simulink model "TCS_straight"  (R2023a)
settings: Solver=VariableStepAuto  StartTime=0.0  StopTime=10.0  RelTol=1e-3
values from neighbouring files (symbols this model uses):
  T1 = 2,T2=2,alpha1=-1.8,alpha2=0.4,A=1    [abs_trial_second_version.m]
undefined symbols (not defined in the file or in its folder): A, alpha1, alpha2, T2, u1, u2, u3
settings Model: Creator=ycmxy  LastModifiedBy=Administrator
settings DebuggingCC: UnconnectedInputMsg=warning  UnconnectedOutputMsg=warning  UnconnectedLineMsg=warning
settings ModelReferenceCC: EnableRefExpFcnMdlSchedulingChecks=on
settings RTWCC: DLArmComputeVersion=19.05

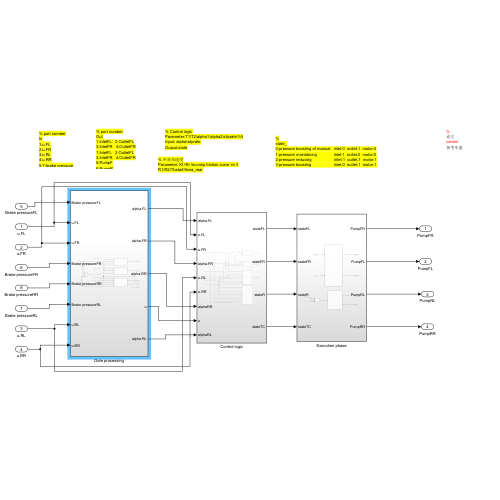
[thumbnail: Simulink's stored preview of the top-level diagram]
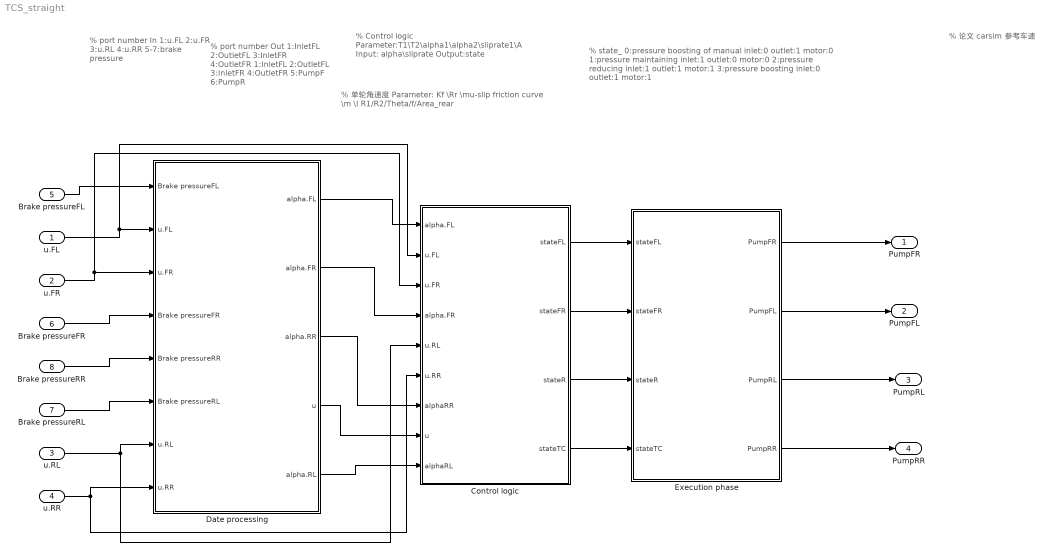
== system TCS_straight ==
  note: % 单轮角速度
      | Parameter: Kf \Rr \mu-slip friction curve \m \I
      | R1/R2/Theta/f/Area_rear
  note: % port number
      | In
      | 1:u.FL
      | 2:u.FR
      | 3:u.RL
      | 4:u.RR
      | 5-7:brake pressure
  note: % Control logic
      | Parameter:T1\T2\alpha1\alpha2\sliprate1\A
      | Input: alpha\sliprate
      | Output:state
  note: %
      | state_
      | 0:pressure boosting of manual inlet:0 outlet:1 motor:0
      | 1:pressure maintaining inlet:1 outlet:0 motor:0
      | 2:pressure reducing inlet:1 outlet:1 motor:1
      | 3:pressure boosting inlet:0 outlet:1 motor:1
  note: % port number
      | Out
      | 1:InletFL 2:OutletFL 3:InletFR 4:OutletFR
      | 1:InletFL 2:OutletFL
      | 3:InletFR 4:OutletFR
      | 5:PumpF
      | 6:PumpR
  note: %
      | 论文
      | carsim
      | 参考车速
  u.FL : Inport
  u.FR : Inport  Port=2
  u.RL : Inport  Port=3
  u.RR : Inport  Port=4
  Brake pressureFL : Inport  Port=5
  Brake pressureFR : Inport  Port=6
  Brake pressureRL : Inport  Port=7
  Brake pressureRR : Inport  Port=8
  Control logic : Subsystem
  Date processing : Subsystem
  Execution phase : Subsystem
  PumpFR : Outport  VectorParamsAs1DForOutWhenUnconnected=off
  PumpFL : Outport  Port=2  VectorParamsAs1DForOutWhenUnconnected=off
  PumpRL : Outport  Port=3  VectorParamsAs1DForOutWhenUnconnected=off
  PumpRR : Outport  Port=4  VectorParamsAs1DForOutWhenUnconnected=off
  wires:
  Execution phase/1(PumpFR) -> PumpFR/1
  u.RR/1 -> Date processing/8(u.RR), Control logic/6(u.RR)
  Brake pressureFL/1 -> Date processing/1(Brake pressureFL)
  Date processing/1(alpha.FL) -> Control logic/1(alpha.FL)
  u.FR/1 -> Control logic/3(u.FR), Date processing/3(u.FR)
  u.FL/1 -> Control logic/2(u.FL), Date processing/2(u.FL)
  Control logic/2(stateFR) -> Execution phase/2(stateFR)
  Date processing/2(alpha.FR) -> Control logic/4(alpha.FR)
  Execution phase/3(PumpRL) -> PumpRL/1
  Brake pressureFR/1 -> Date processing/4(Brake pressureFR)
  Control logic/3(stateR) -> Execution phase/3(stateR)
  Date processing/4(u) -> Control logic/8(u)
  Date processing/3(alpha.RR) -> Control logic/7(alphaRR)
  Brake pressureRR/1 -> Date processing/5(Brake pressureRR)
  u.RL/1 -> Control logic/5(u.RL), Date processing/7(u.RL)
  Control logic/1(stateFL) -> Execution phase/1(stateFL)
  Execution phase/4(PumpRR) -> PumpRR/1
  Brake pressureRL/1 -> Date processing/6(Brake pressureRL)
  Execution phase/2(PumpFL) -> PumpFL/1
  Date processing/5(alpha.RL) -> Control logic/9(alphaRL)
  Control logic/4(stateTC) -> Execution phase/4(stateTC)

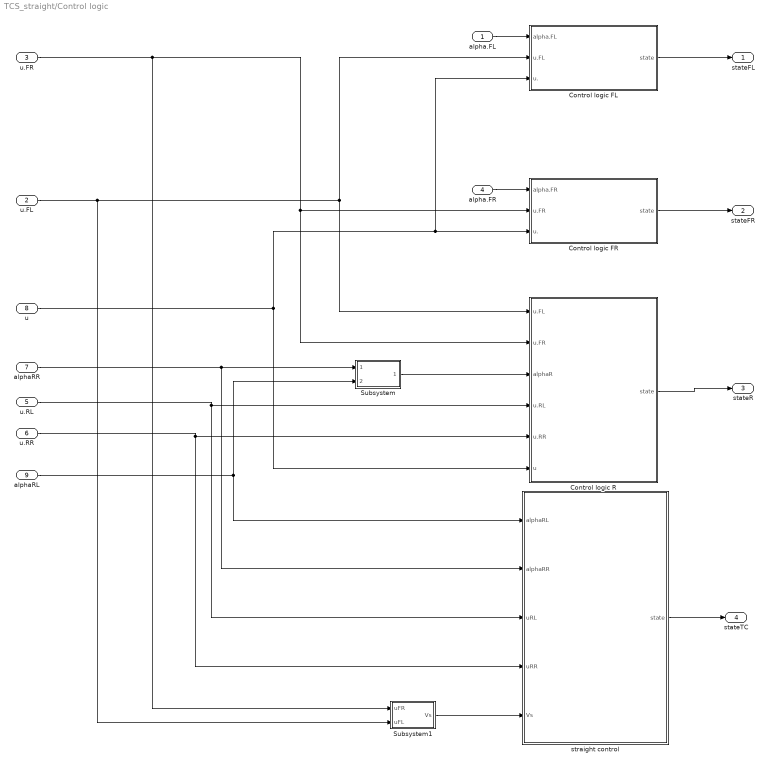
== system TCS_straight/Control logic ==
  alpha.FL : Inport
  u.FL : Inport  Port=2
  u.FR : Inport  Port=3
  alpha.FR : Inport  Port=4
  u.RL : Inport  Port=5
  u.RR : Inport  Port=6
  alphaRR : Inport  Port=7
  u : Inport  Port=8
  alphaRL : Inport  Port=9
  Control logic FL : Subsystem
  Control logic FR : Subsystem
  Control logic R : Subsystem
  Subsystem : Subsystem
  Subsystem1 : Subsystem
  straight control : Subsystem
  stateFL : Outport
  stateFR : Outport  Port=2
  stateR : Outport  Port=3
  stateTC : Outport  Port=4
  wires:
  u.FL/1 -> Subsystem1/2(uFL), Control logic FL/2(u.FL), Control logic R/1(u.FL)
  u.RR/1 -> straight control/4(uRR), Control logic R/5(u.RR)
  Control logic FR/1(state) -> stateFR/1
  u.FR/1 -> Subsystem1/1(uFR), Control logic R/2(u.FR), Control logic FR/2(u.FR)
  alpha.FR/1 -> Control logic FR/1(alpha.FR)
  alpha.FL/1 -> Control logic FL/1(alpha.FL)
  Control logic R/1(state) -> stateR/1
  Control logic FL/1(state) -> stateFL/1
  u.RL/1 -> straight control/3(uRL), Control logic R/4(u.RL)
  u/1 -> Control logic FR/3(u.), Control logic FL/3(u.), Control logic R/6(u)
  alphaRR/1 -> straight control/2(alphaRR), Subsystem/1(alphaRR)
  alphaRL/1 -> straight control/1(alphaRL), Subsystem/2(alphaRL)
  Subsystem/1(alphaR) -> Control logic R/3(alphaR)
  Subsystem1/1(Vs) -> straight control/5(Vs)
  straight control/1(state) -> stateTC/1

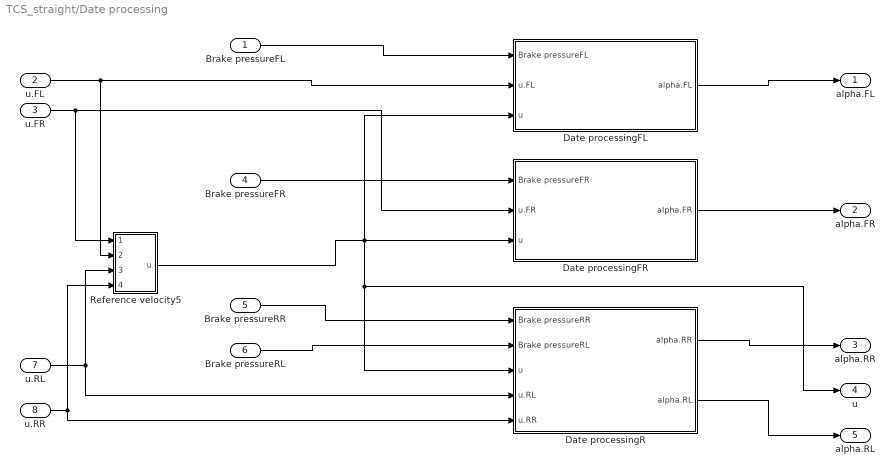
== system TCS_straight/Date processing ==
  Brake pressureFL : Inport
  u.FL : Inport  Port=2
  u.FR : Inport  Port=3
  Brake pressureFR : Inport  Port=4
  Brake pressureRR : Inport  Port=5
  Brake pressureRL : Inport  Port=6
  u.RL : Inport  Port=7
  u.RR : Inport  Port=8
  Date processingFL : Subsystem
  Date processingFR : Subsystem
  Date processingR : Subsystem
  Reference velocity5 : Subsystem
  alpha.FL : Outport
  alpha.FR : Outport  Port=2
  alpha.RR : Outport  Port=3
  u : Outport  Port=4
  alpha.RL : Outport  Port=5
  wires:
  Date processingR/1(alpha.RR) -> alpha.RR/1
  u.FL/1 -> Reference velocity5/2(u.FL), Date processingFL/2(u.FL)
  Brake pressureRR/1 -> Date processingR/1(Brake pressureRR)
  u.FR/1 -> Reference velocity5/1(u.FR), Date processingFR/2(u.FR)
  Brake pressureFL/1 -> Date processingFL/1(Brake pressureFL)
  u.RL/1 -> Reference velocity5/3(u.RL), Date processingR/4(u.RL)
  Date processingFL/1(alpha.FL) -> alpha.FL/1
  Date processingFR/1(alpha.FR) -> alpha.FR/1
  Brake pressureFR/1 -> Date processingFR/1(Brake pressureFR)
  Brake pressureRL/1 -> Date processingR/2(Brake pressureRL)
  u.RR/1 -> Reference velocity5/4(u.RR), Date processingR/5(u.RR)
  Reference velocity5/1(u) -> Date processingFL/3(u), Date processingFR/3(u), u/1, Date processingR/3(u)
  Date processingR/2(alpha.RL) -> alpha.RL/1

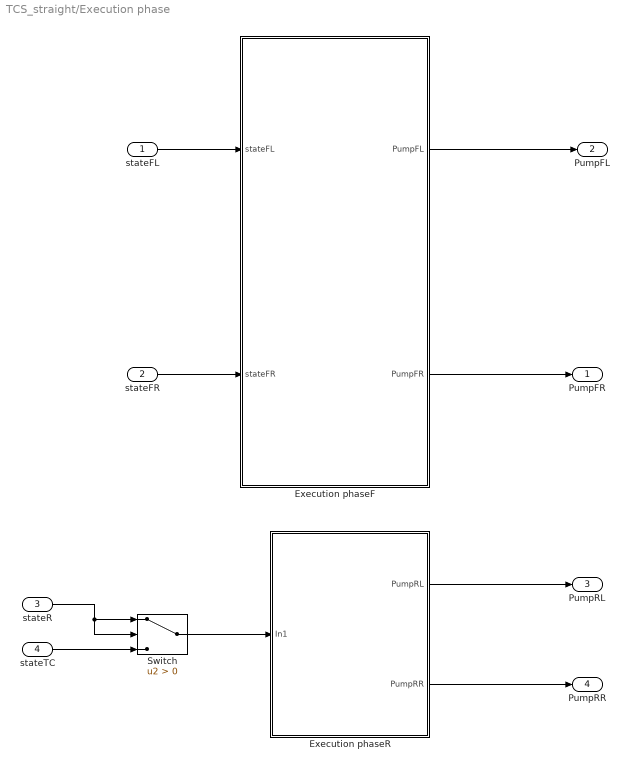
== system TCS_straight/Execution phase ==
  stateFL : Inport
  stateFR : Inport  Port=2
  stateR : Inport  Port=3
  stateTC : Inport  Port=4
  Execution phaseF : Subsystem
  Execution phaseR : Subsystem
  Switch : Switch  Criteria=u2 > Threshold  SaturateOnIntegerOverflow=off  InputSameDT=off
  PumpFR : Outport
  PumpFL : Outport  Port=2
  PumpRL : Outport  Port=3
  PumpRR : Outport  Port=4
  wires:
  stateFL/1 -> Execution phaseF/1(stateFL)
  stateFR/1 -> Execution phaseF/2(stateFR)
  Execution phaseR/1(PumpRL) -> PumpRL/1
  Execution phaseF/1(PumpFL) -> PumpFL/1
  Execution phaseF/2(PumpFR) -> PumpFR/1
  Execution phaseR/2(PumpRR) -> PumpRR/1
  stateR/1 -> Switch/1, Switch/2
  stateTC/1 -> Switch/3
  Switch/1 -> Execution phaseR/1(In1)

== system TCS_straight/Control logic/Control logic FL ==
  alpha.FL : Inport
  u.FL : Inport  Port=2
  u. : Inport  Port=3
  FL : Stateflow chart  TreatAsAtomicUnit=on
  Gain : Gain  Gain=0.8
  state : Outport  VectorParamsAs1DForOutWhenUnconnected=off
  wires:
  alpha.FL/1 -> FL/1(alpha)
  FL/1(state) -> state/1
  u.FL/1 -> FL/2(omegaR)
  Gain/1 -> FL/3(sliprate1)
  u./1 -> Gain/1

== system TCS_straight/Control logic/Control logic FR ==
  alpha.FR : Inport
  u.FR : Inport  Port=2
  u. : Inport  Port=3
  FR : Stateflow chart  TreatAsAtomicUnit=on
  Gain : Gain  Gain=0.8
  state : Outport  VectorParamsAs1DForOutWhenUnconnected=off
  wires:
  alpha.FR/1 -> FR/1(alpha)
  FR/1(state) -> state/1
  u.FR/1 -> FR/2(omegaR)
  Gain/1 -> FR/3(sliprate1)
  u./1 -> Gain/1

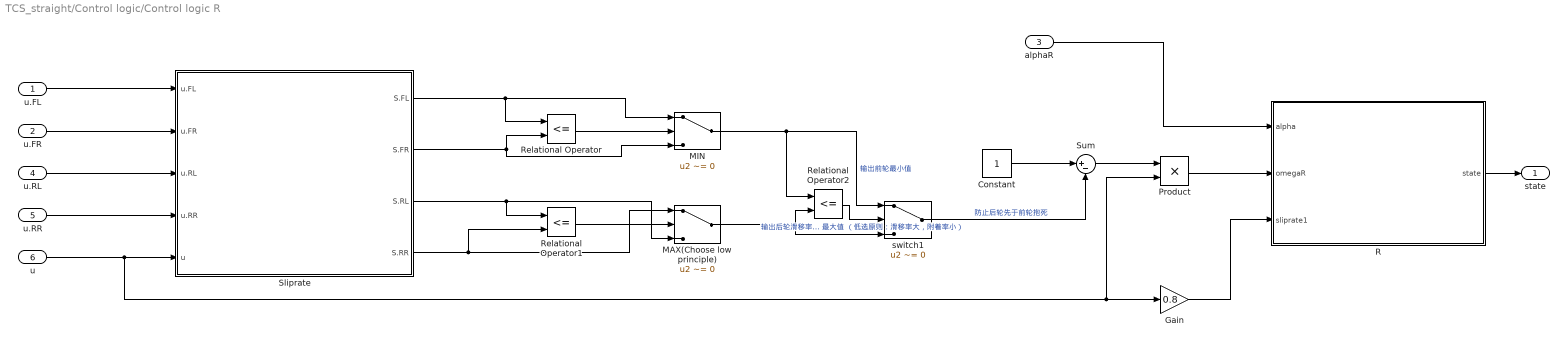
== system TCS_straight/Control logic/Control logic R ==
  u.FL : Inport
  u.FR : Inport  Port=2
  alphaR : Inport  Port=3
  u.RL : Inport  Port=4
  u.RR : Inport  Port=5
  u : Inport  Port=6
  Constant : Constant
  Gain : Gain  Gain=0.8
  MAX(Choose low principle) : Switch  Criteria=u2 ~= 0  SaturateOnIntegerOverflow=off  InputSameDT=off
  MIN : Switch  Criteria=u2 ~= 0  SaturateOnIntegerOverflow=off  InputSameDT=off
  Product : Product
  R : Stateflow chart  TreatAsAtomicUnit=on
  Relational Operator : RelationalOperator  Operator=<=  OutDataTypeStr=boolean  RndMeth=Simplest  InputSameDT=off
  Relational Operator1 : RelationalOperator  Operator=<=  OutDataTypeStr=boolean  RndMeth=Simplest  InputSameDT=off
  Relational Operator2 : RelationalOperator  Operator=<=  OutDataTypeStr=boolean  RndMeth=Simplest  InputSameDT=off
  Sliprate : Subsystem
  Sum : Sum  Inputs=|+-
  switch1 : Switch  Criteria=u2 ~= 0  SaturateOnIntegerOverflow=off  InputSameDT=off
  state : Outport  VectorParamsAs1DForOutWhenUnconnected=off
  wires:
  MAX(Choose low principle)/1 -> switch1/3, Relational Operator2/2  "输出后轮滑移率 最大值 （低选原则：滑移率大，附着率小）"
  switch1/1 -> Sum/2  "防止后轮先于前轮抱死"
  u.FR/1 -> Sliprate/2(u.FR)
  Sliprate/2(S.FR) -> MIN/3, Relational Operator/2
  Sliprate/1(S.FL) -> Relational Operator/1, MIN/1
  Relational Operator2/1 -> switch1/2
  Relational Operator/1 -> MIN/2
  MIN/1 -> Relational Operator2/1, switch1/1  "输出前轮最小值"
  Sliprate/4(S.RR) -> MAX(Choose low principle)/1, Relational Operator1/2
  Relational Operator1/1 -> MAX(Choose low principle)/2
  u.RL/1 -> Sliprate/3(u.RL)
  Sliprate/3(S.RL) -> Relational Operator1/1, MAX(Choose low principle)/3
  u/1 -> Product/2, Gain/1, Sliprate/5(u)
  alphaR/1 -> R/1(alpha)
  u.FL/1 -> Sliprate/1(u.FL)
  R/1(state) -> state/1
  u.RR/1 -> Sliprate/4(u.RR)
  Gain/1 -> R/3(sliprate1)
  Constant/1 -> Sum/1
  Product/1 -> R/2(omegaR)
  Sum/1 -> Product/1

== system TCS_straight/Control logic/Subsystem ==
  alphaRR : Inport
  alphaRL : Inport  Port=2
  Multiply : Gain  Gain=1/2
  Sum : Sum  Inputs=|++
  alphaR : Outport
  wires:
  alphaRR/1 -> Sum/1
  alphaRL/1 -> Sum/2
  Sum/1 -> Multiply/1
  Multiply/1 -> alphaR/1

== system TCS_straight/Control logic/Subsystem1 ==
  uFR : Inport
  uFL : Inport  Port=2
  Multiply : Gain  Gain=1/2
  Sum : Sum  Inputs=|++
  Vs : Outport
  wires:
  uFR/1 -> Sum/1
  uFL/1 -> Sum/2
  Sum/1 -> Multiply/1
  Multiply/1 -> Vs/1

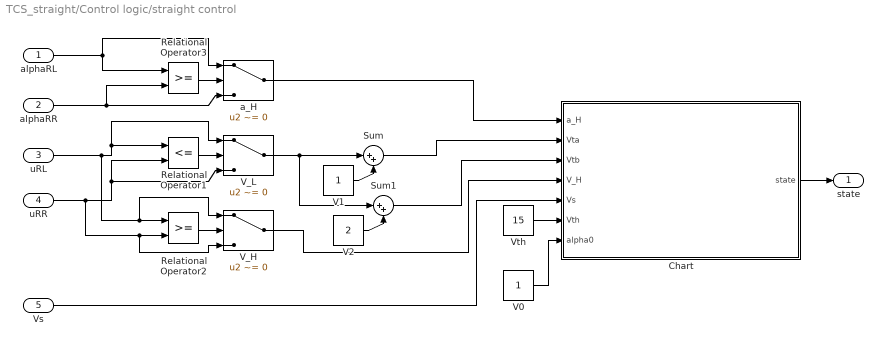
== system TCS_straight/Control logic/straight control ==
  alphaRL : Inport
  alphaRR : Inport  Port=2
  uRL : Inport  Port=3
  uRR : Inport  Port=4
  Vs : Inport  Port=5
  Chart : Stateflow chart  TreatAsAtomicUnit=on
  Relational Operator1 : RelationalOperator  Operator=<=  OutDataTypeStr=boolean  RndMeth=Simplest  InputSameDT=off
  Relational Operator2 : RelationalOperator  OutDataTypeStr=boolean  RndMeth=Simplest  InputSameDT=off
  Relational Operator3 : RelationalOperator  OutDataTypeStr=boolean  RndMeth=Simplest  InputSameDT=off
  Sum : Sum  Inputs=|++
  Sum1 : Sum  Inputs=|++
  V0 : Constant
  V1 : Constant
  V2 : Constant  Value=2
  V_H : Switch  Criteria=u2 ~= 0  SaturateOnIntegerOverflow=off  InputSameDT=off
  V_L : Switch  Criteria=u2 ~= 0  SaturateOnIntegerOverflow=off  InputSameDT=off
  Vth : Constant  Value=15
  a_H : Switch  Criteria=u2 ~= 0  SaturateOnIntegerOverflow=off  InputSameDT=off
  state : Outport
  wires:
  Relational Operator3/1 -> a_H/2
  alphaRL/1 -> Relational Operator3/1, a_H/1
  alphaRR/1 -> a_H/3, Relational Operator3/2
  Relational Operator1/1 -> V_L/2
  uRL/1 -> V_H/1, Relational Operator2/1, V_L/1, Relational Operator1/1
  uRR/1 -> V_H/3, Relational Operator2/2, V_L/3, Relational Operator1/2
  Relational Operator2/1 -> V_H/2
  V1/1 -> Sum/2
  V_L/1 -> Sum/1, Sum1/1
  V2/1 -> Sum1/2
  Sum/1 -> Chart/2(Vta)
  Sum1/1 -> Chart/3(Vtb)
  Vs/1 -> Chart/5(Vs)
  V_H/1 -> Chart/4(V_H)
  a_H/1 -> Chart/1(a_H)
  Chart/1(state) -> state/1
  Vth/1 -> Chart/6(Vth)
  V0/1 -> Chart/7(alpha0)

== system TCS_straight/Date processing/Date processingFL ==
  Brake pressureFL : Inport
  u.FL : Inport  Port=2
  u : Inport  Port=3
  Tire angular velocity.FL : Subsystem
  alpha.FL : Outport
  wires:
  Tire angular velocity.FL/1(alpha.FL) -> alpha.FL/1
  u/1 -> Tire angular velocity.FL/3(u)
  Brake pressureFL/1 -> Tire angular velocity.FL/1(Brakepressure)
  u.FL/1 -> Tire angular velocity.FL/2(u.FL)

== system TCS_straight/Date processing/Date processingFR ==
  Brake pressureFR : Inport
  u.FR : Inport  Port=2
  u : Inport  Port=3
  Tire angular velocity.FR : Subsystem
  alpha.FR : Outport
  wires:
  u.FR/1 -> Tire angular velocity.FR/1(u.FR)
  Tire angular velocity.FR/1(alpha.FR) -> alpha.FR/1
  Brake pressureFR/1 -> Tire angular velocity.FR/3(Brake pressure)
  u/1 -> Tire angular velocity.FR/2(u)

== system TCS_straight/Date processing/Date processingR ==
  Brake pressureRR : Inport
  Brake pressureRL : Inport  Port=2
  u : Inport  Port=3
  u.RL : Inport  Port=4
  u.RR : Inport  Port=5
  Tire angular velocity.R : Subsystem
  Tire angular velocity.R1 : Subsystem
  alpha.RR : Outport
  alpha.RL : Outport  Port=2
  wires:
  Tire angular velocity.R/1(alpha.RR) -> alpha.RR/1
  u.RR/1 -> Tire angular velocity.R/3(u.RR)
  Brake pressureRR/1 -> Tire angular velocity.R/1(Brake pressureRR)
  Tire angular velocity.R1/1(alpha.RR) -> alpha.RL/1
  u/1 -> Tire angular velocity.R/2(u), Tire angular velocity.R1/2(u)
  u.RL/1 -> Tire angular velocity.R1/3(u.RL)
  Brake pressureRL/1 -> Tire angular velocity.R1/1(Brake pressureRR)

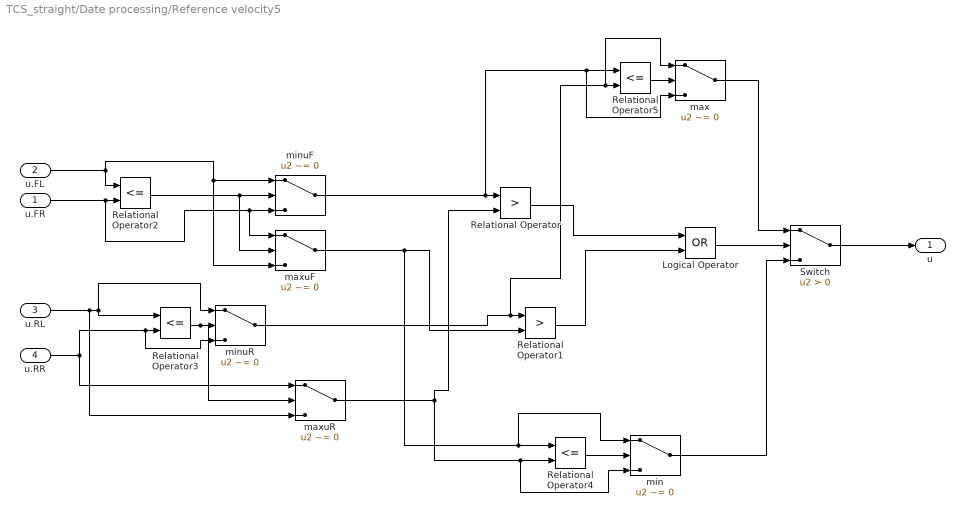
== system TCS_straight/Date processing/Reference velocity5 ==
  u.FR : Inport
  u.FL : Inport  Port=2
  u.RL : Inport  Port=3
  u.RR : Inport  Port=4
  Logical Operator : Logic  Operator=OR  AllPortsSameDT=off  OutDataTypeStr=boolean
  Relational Operator : RelationalOperator  Operator=>  OutDataTypeStr=boolean  RndMeth=Simplest  InputSameDT=off
  Relational Operator1 : RelationalOperator  Operator=>  OutDataTypeStr=boolean  RndMeth=Simplest  InputSameDT=off
  Relational Operator{2..5} (4 alike) : RelationalOperator  Operator=<=  OutDataTypeStr=boolean  RndMeth=Simplest  InputSameDT=off
  Switch : Switch  Criteria=u2 > Threshold  SaturateOnIntegerOverflow=off  InputSameDT=off
  max : Switch  Criteria=u2 ~= 0  SaturateOnIntegerOverflow=off  InputSameDT=off
  maxuF : Switch  Criteria=u2 ~= 0  SaturateOnIntegerOverflow=off  InputSameDT=off
  maxuR : Switch  Criteria=u2 ~= 0  SaturateOnIntegerOverflow=off  InputSameDT=off
  min : Switch  Criteria=u2 ~= 0  SaturateOnIntegerOverflow=off  InputSameDT=off
  minuF : Switch  Criteria=u2 ~= 0  SaturateOnIntegerOverflow=off  InputSameDT=off
  minuR : Switch  Criteria=u2 ~= 0  SaturateOnIntegerOverflow=off  InputSameDT=off
  u : Outport  VectorParamsAs1DForOutWhenUnconnected=off
  wires:
  u.FR/1 -> maxuF/1, minuF/3, Relational Operator2/2
  u.FL/1 -> minuF/1, maxuF/3, Relational Operator2/1
  u.RL/1 -> maxuR/3, minuR/1, Relational Operator3/1
  u.RR/1 -> maxuR/1, minuR/3, Relational Operator3/2
  minuF/1 -> max/3, Relational Operator5/1, Relational Operator/1
  maxuR/1 -> min/3, Relational Operator4/2, Relational Operator/2
  minuR/1 -> max/1, Relational Operator5/2, Relational Operator1/1
  maxuF/1 -> min/1, Relational Operator4/1, Relational Operator1/2
  Relational Operator/1 -> Logical Operator/1
  Relational Operator1/1 -> Logical Operator/2
  Logical Operator/1 -> Switch/2
  min/1 -> Switch/3
  max/1 -> Switch/1
  Switch/1 -> u/1
  Relational Operator2/1 -> minuF/2, maxuF/2
  Relational Operator3/1 -> maxuR/2, minuR/2
  Relational Operator4/1 -> min/2
  Relational Operator5/1 -> max/2

== system TCS_straight/Execution phase/Execution phaseF ==
  stateFL : Inport
  stateFR : Inport  Port=2
  Execution phaseFL : Stateflow chart  TreatAsAtomicUnit=on
  Execution phaseFR : Stateflow chart  TreatAsAtomicUnit=on
  PumpFL : Outport  VectorParamsAs1DForOutWhenUnconnected=off
  PumpFR : Outport  Port=2  VectorParamsAs1DForOutWhenUnconnected=off
  wires:
  stateFL/1 -> Execution phaseFL/1(state)
  stateFR/1 -> Execution phaseFR/1(state)
  Execution phaseFL/1(Pump) -> PumpFL/1
  Execution phaseFR/1(Pump) -> PumpFR/1

== system TCS_straight/Execution phase/Execution phaseR ==
  In1 : Inport
  Execution phaseRL : Stateflow chart  TreatAsAtomicUnit=on
  Execution phaseRR : Stateflow chart  TreatAsAtomicUnit=on
  PumpRL : Outport  VectorParamsAs1DForOutWhenUnconnected=off
  PumpRR : Outport  Port=2  VectorParamsAs1DForOutWhenUnconnected=off
  wires:
  In1/1 -> Execution phaseRR/1(state), Execution phaseRL/1(state)
  Execution phaseRR/1(Pump) -> PumpRR/1
  Execution phaseRL/1(Pump) -> PumpRL/1

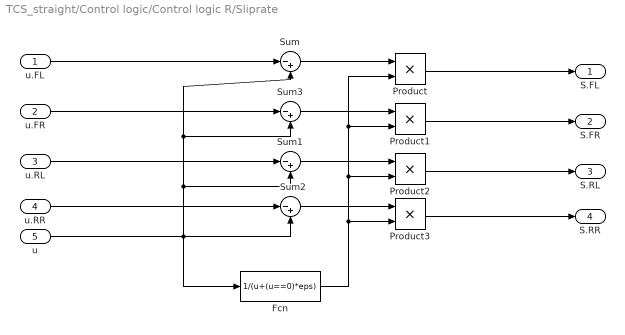
== system TCS_straight/Control logic/Control logic R/Sliprate ==
  u.FL : Inport
  u.FR : Inport  Port=2
  u.RL : Inport  Port=3
  u.RR : Inport  Port=4
  u : Inport  Port=5
  Fcn : Fcn  Expr=1/(u+(u==0)*eps)
  Product{,1..3} (4 alike) : Product
  Sum{,1..3} (4 alike) : Sum  Inputs=|-+
  S.FL : Outport  VectorParamsAs1DForOutWhenUnconnected=off
  S.FR : Outport  Port=2  VectorParamsAs1DForOutWhenUnconnected=off
  S.RL : Outport  Port=3  VectorParamsAs1DForOutWhenUnconnected=off
  S.RR : Outport  Port=4  VectorParamsAs1DForOutWhenUnconnected=off
  wires:
  Sum2/1 -> Product3/1
  Sum/1 -> Product/1
  Fcn/1 -> Product3/2, Product2/2, Product1/2, Product/2
  Sum1/1 -> Product2/1
  Sum3/1 -> Product1/1
  u/1 -> Sum2/2, Fcn/1, Sum1/2, Sum3/2, Sum/2
  u.RL/1 -> Sum1/1
  u.RR/1 -> Sum2/1
  Product2/1 -> S.RL/1
  Product3/1 -> S.RR/1
  Product/1 -> S.FL/1
  Product1/1 -> S.FR/1
  u.FL/1 -> Sum/1
  u.FR/1 -> Sum3/1

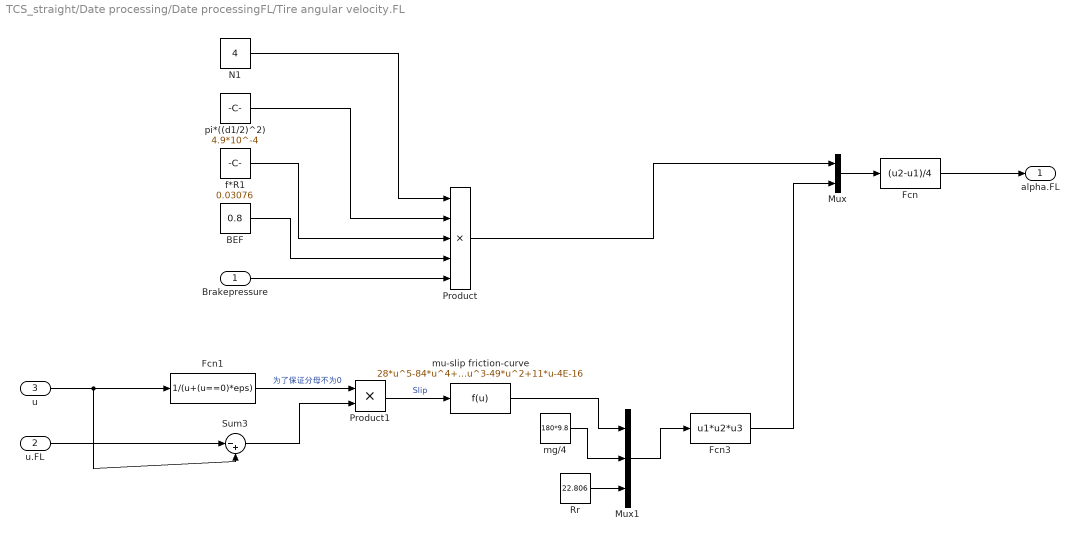
== system TCS_straight/Date processing/Date processingFL/Tire angular velocity.FL ==
  Brakepressure : Inport
  u.FL : Inport  Port=2
  u : Inport  Port=3
  BEF : Constant  Value=0.8
  Fcn : Fcn  Expr=(u2-u1)/4
  Fcn1 : Fcn  Expr=1/(u+(u==0)*eps)
  Fcn3 : Fcn  Expr=u1*u2*u3
  Mux : Mux  Inputs=2
  Mux1 : Mux  Inputs=3
  N1 : Constant  Value=4
  Product : Product  Inputs=5
  Product1 : Product
  Rr : Constant  Value=22.806
  Sum3 : Sum  Inputs=|-+
  f*R1 : Constant  Value=0.03076
  mg/4 : Constant  Value=180*9.8
  mu-slip friction-curve : Fcn  Expr=28*u^5-84*u^4+94.5*u^3-49*u^2+11*u-4E-16
  pi*((d1/2)^2) : Constant  Value=4.9*10^-4
  alpha.FL : Outport  VectorParamsAs1DForOutWhenUnconnected=off
  wires:
  mu-slip friction-curve/1 -> Mux1/1
  Sum3/1 -> Product1/2
  u.FL/1 -> Sum3/1
  u/1 -> Fcn1/1, Sum3/2
  Fcn1/1 -> Product1/1  "为了保证分母不为0"
  Product1/1 -> mu-slip friction-curve/1  "Slip"
  N1/1 -> Product/1
  pi*((d1/2)^2)/1 -> Product/2
  f*R1/1 -> Product/3
  BEF/1 -> Product/4
  Brakepressure/1 -> Product/5
  Mux/1 -> Fcn/1
  Product/1 -> Mux/1
  Fcn/1 -> alpha.FL/1
  Mux1/1 -> Fcn3/1
  mg/4/1 -> Mux1/2
  Rr/1 -> Mux1/3
  Fcn3/1 -> Mux/2

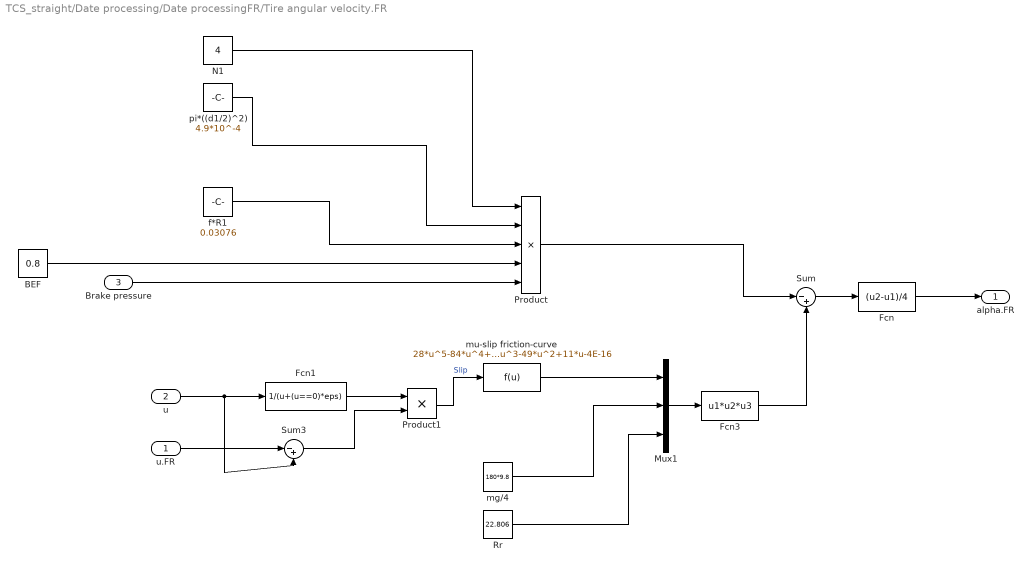
== system TCS_straight/Date processing/Date processingFR/Tire angular velocity.FR ==
  u.FR : Inport
  u : Inport  Port=2
  Brake pressure : Inport  Port=3
  BEF : Constant  Value=0.8
  Fcn : Fcn  Expr=(u2-u1)/4
  Fcn1 : Fcn  Expr=1/(u+(u==0)*eps)
  Fcn3 : Fcn  Expr=u1*u2*u3
  Mux1 : Mux  Inputs=3
  N1 : Constant  Value=4
  Product : Product  Inputs=5
  Product1 : Product
  Rr : Constant  Value=22.806
  Sum : Sum  Inputs=|-+
  Sum3 : Sum  Inputs=|-+
  f*R1 : Constant  Value=0.03076
  mg/4 : Constant  Value=180*9.8
  mu-slip friction-curve : Fcn  Expr=28*u^5-84*u^4+94.5*u^3-49*u^2+11*u-4E-16
  pi*((d1/2)^2) : Constant  Value=4.9*10^-4
  alpha.FR : Outport  VectorParamsAs1DForOutWhenUnconnected=off
  wires:
  Fcn1/1 -> Product1/1
  u/1 -> Fcn1/1, Sum3/2
  u.FR/1 -> Sum3/1
  Sum3/1 -> Product1/2
  Sum/1 -> Fcn/1
  BEF/1 -> Product/4
  f*R1/1 -> Product/3
  pi*((d1/2)^2)/1 -> Product/2
  N1/1 -> Product/1
  Brake pressure/1 -> Product/5
  Product/1 -> Sum/1
  Fcn3/1 -> Sum/2
  Mux1/1 -> Fcn3/1
  mu-slip friction-curve/1 -> Mux1/1
  Product1/1 -> mu-slip friction-curve/1  "Slip"
  mg/4/1 -> Mux1/2
  Rr/1 -> Mux1/3
  Fcn/1 -> alpha.FR/1

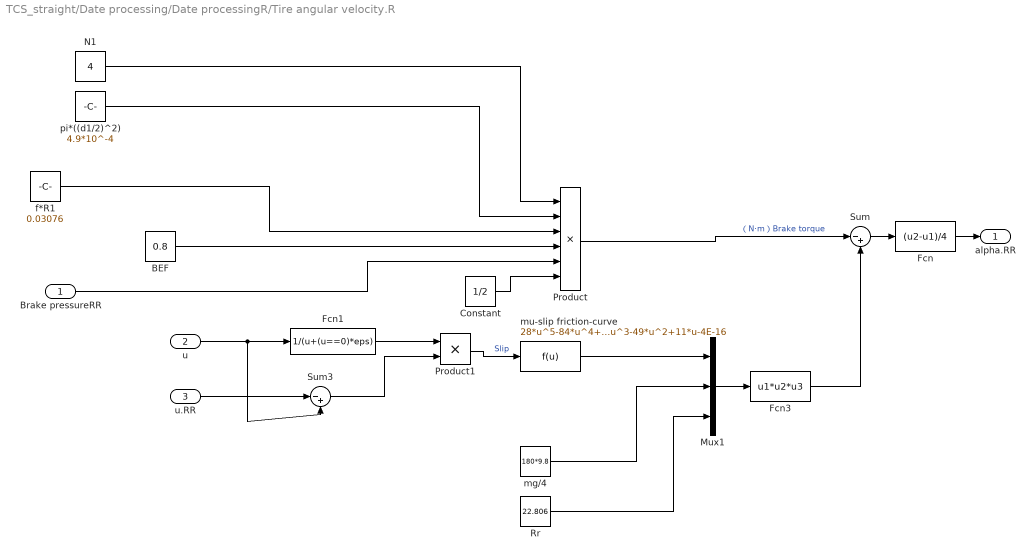
== system TCS_straight/Date processing/Date processingR/Tire angular velocity.R ==
  Brake pressureRR : Inport
  u : Inport  Port=2
  u.RR : Inport  Port=3
  BEF : Constant  Value=0.8
  Constant : Constant  Value=1/2
  Fcn : Fcn  Expr=(u2-u1)/4
  Fcn1 : Fcn  Expr=1/(u+(u==0)*eps)
  Fcn3 : Fcn  Expr=u1*u2*u3
  Mux1 : Mux  Inputs=3
  N1 : Constant  Value=4
  Product : Product  Inputs=6
  Product1 : Product
  Rr : Constant  Value=22.806
  Sum : Sum  Inputs=|-+
  Sum3 : Sum  Inputs=|-+
  f*R1 : Constant  Value=0.03076
  mg/4 : Constant  Value=180*9.8
  mu-slip friction-curve : Fcn  Expr=28*u^5-84*u^4+94.5*u^3-49*u^2+11*u-4E-16
  pi*((d1/2)^2) : Constant  Value=4.9*10^-4
  alpha.RR : Outport  VectorParamsAs1DForOutWhenUnconnected=off
  wires:
  Sum3/1 -> Product1/2
  u.RR/1 -> Sum3/1
  u/1 -> Sum3/2, Fcn1/1
  Fcn1/1 -> Product1/1
  Product/1 -> Sum/1  "（N·m）Brake torque"
  BEF/1 -> Product/4
  N1/1 -> Product/1
  f*R1/1 -> Product/3
  pi*((d1/2)^2)/1 -> Product/2
  Brake pressureRR/1 -> Product/5
  Constant/1 -> Product/6
  Sum/1 -> Fcn/1
  Fcn/1 -> alpha.RR/1
  mu-slip friction-curve/1 -> Mux1/1
  Mux1/1 -> Fcn3/1
  mg/4/1 -> Mux1/2
  Product1/1 -> mu-slip friction-curve/1  "Slip"
  Rr/1 -> Mux1/3
  Fcn3/1 -> Sum/2

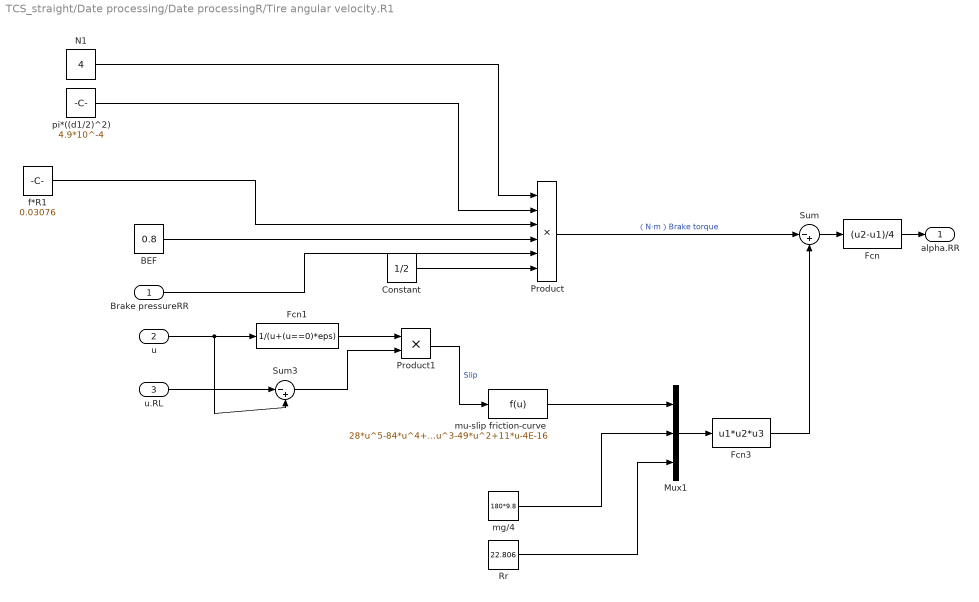
== system TCS_straight/Date processing/Date processingR/Tire angular velocity.R1 ==
  Brake pressureRR : Inport
  u : Inport  Port=2
  u.RL : Inport  Port=3
  BEF : Constant  Value=0.8
  Constant : Constant  Value=1/2
  Fcn : Fcn  Expr=(u2-u1)/4
  Fcn1 : Fcn  Expr=1/(u+(u==0)*eps)
  Fcn3 : Fcn  Expr=u1*u2*u3
  Mux1 : Mux  Inputs=3
  N1 : Constant  Value=4
  Product : Product  Inputs=6
  Product1 : Product
  Rr : Constant  Value=22.806
  Sum : Sum  Inputs=|-+
  Sum3 : Sum  Inputs=|-+
  f*R1 : Constant  Value=0.03076
  mg/4 : Constant  Value=180*9.8
  mu-slip friction-curve : Fcn  Expr=28*u^5-84*u^4+94.5*u^3-49*u^2+11*u-4E-16
  pi*((d1/2)^2) : Constant  Value=4.9*10^-4
  alpha.RR : Outport  VectorParamsAs1DForOutWhenUnconnected=off
  wires:
  Sum3/1 -> Product1/2
  u.RL/1 -> Sum3/1
  u/1 -> Sum3/2, Fcn1/1
  Fcn1/1 -> Product1/1
  N1/1 -> Product/1
  Product/1 -> Sum/1  "（N·m）Brake torque"
  pi*((d1/2)^2)/1 -> Product/2
  f*R1/1 -> Product/3
  BEF/1 -> Product/4
  Constant/1 -> Product/6
  Brake pressureRR/1 -> Product/5
  Rr/1 -> Mux1/3
  mu-slip friction-curve/1 -> Mux1/1
  Mux1/1 -> Fcn3/1
  mg/4/1 -> Mux1/2
  Fcn3/1 -> Sum/2
  Product1/1 -> mu-slip friction-curve/1  "Slip"
  Sum/1 -> Fcn/1
  Fcn/1 -> alpha.RR/1

== stateflow chart TCS_straight/Control logic/Control logic R/R ==
  state state_ [group]
    0:pressure boosting of manual
    1:pressure maintaining
    2:pressure reducing
    3:pressure boosting
    Parameter:
    T1 T2
    alpha1\alpha2\sliprate1\A
    Input: alpha\sliprate
    Output:state
  state phase2     %state pressure reducing
    state phase3_1
      en:
      state= 2;
    state phase3_2
      en:
      state= 1;
    (default) -> phase3_1
    phase3_1 -> phase3_2 : after(T1,sec)
    phase3_2 -> phase3_1 : after(T1,sec)
  state phase0
    en:
    state= 0;
  state phase1
    en:
    state= 1;
  state phase4_2     %state pressure reducing
    state phase4_2_1
      en:
      state= 2;
    state phase4_2_2
      en:
      state= 1;
    (default) -> phase4_2_1
    phase4_2_1 -> phase4_2_2 : after(T1,sec)
    phase4_2_2 -> phase4_2_1 : after(T1,sec)
  state phase4_1     %state pressure boosting
    state phase4_1_1
      en:
      state= 3;
    state phase4_1_2
      en:
      state= 1;
    (default) -> phase4_1_1
    phase4_1_1 -> phase4_1_2 : after(T2,sec)
    phase4_1_2 -> phase4_1_1 : after(T2,sec)
  state phase3
    en:
    state= 1;
  state phase4_ 1 2 3: [group]
    路面附着系数识别阶段
  state phase4_3
    en:
    state= 1;
  state phase5     %state pressure boosting
    state phase5_1
      en:
      state= 3;
    state phase5_2
      en:
      state= 1;
    (default) -> phase5_1
    phase5_1 -> phase5_2 : after(T2,sec)
    phase5_2 -> phase5_1 : after(T2,sec)
  state phase5_ [group]
    第一周期结束
  (default) -> phase0
  phase0 -> phase1 : [alpha<alpha1]
      | %开始作用
  phase1 -> phase2     %state pressure reducing : [omegaR<sliprate1]
  phase5     %state pressure boosting -> phase1 : [alpha<alpha1]
  phase2     %state pressure reducing -> phase3 : [alpha>alpha1]
  phase3 -> (junction 25)
  (junction 25) -> phase4_1     %state pressure boosting [order 3] : [alpha>A]
  (junction 25) -> phase4_2     %state pressure reducing [order 2] : [alpha<alpha2]
  (junction 25) -> phase4_3 [order 1] : [alpha2<alpha<A]
  phase4_2     %state pressure reducing -> phase4_3 : [alpha>alpha2]
  phase4_1     %state pressure boosting -> phase4_3 : [alpha<A]
  phase4_3 -> phase5     %state pressure boosting : [alpha<alpha2]
  data: alpha input; alpha1 parameter; alpha2 parameter; omegaR input; A parameter; T1 parameter; T2 parameter; state output; sliprate1 input

== stateflow chart TCS_straight/Control logic/Control logic FL/FL ==
  state state_ [group]
    0:pressure boosting of manual
    1:pressure maintaining
    2:pressure reducing
    3:pressure boosting
    Parameter:
    T1 T2
    alpha1\alpha2\sliprate1\A
    Input: alpha\sliprate
    Output:state
  state phase2     %state pressure reducing
    state phase2_1
      en:
      state= 2;
    state phase2_2
      en:
      state= 1;
    (default) -> phase2_1
    phase2_1 -> phase2_2 : after(T1,sec)
    phase2_2 -> phase2_1 : after(T1,sec)
  state phase0
    en:
    state= 0;
  state phase1
    en:
    state= 1;
  state phase4_2     %state pressure reducing
    state phase4_2_1
      en:
      state= 2;
    state phase4_2_2
      en:
      state= 1;
    (default) -> phase4_2_1
    phase4_2_1 -> phase4_2_2 : after(T1,sec)
    phase4_2_2 -> phase4_2_1 : after(T1,sec)
  state phase4_1     %state pressure boosting
    state phase4_1_1
      en:
      state= 3;
    state phase4_1_2
      en:
      state= 1;
    (default) -> phase4_1_1
    phase4_1_1 -> phase4_1_2 : after(T2,sec)
    phase4_1_2 -> phase4_1_1 : after(T2,sec)
  state phase3
    en:
    state= 1;
  state phase4_ 1 2 3: [group]
    路面附着系数识别阶段
  state phase4_3
    en:
    state= 1;
  state phase5     %state pressure boosting
    state phase5_1
      en:
      state= 3;
    state phase5_2
      en:
      state= 1;
    (default) -> phase5_1
    phase5_1 -> phase5_2 : after(T2,sec)
    phase5_2 -> phase5_1 : after(T2,sec)
  state phase5_ [group]
    第一周期结束
  (default) -> phase0
  phase0 -> phase1 : [alpha<alpha1]
      | %开始作用
  phase1 -> phase2     %state pressure reducing : [omegaR<sliprate1]
  phase5     %state pressure boosting -> phase1 : [alpha<alpha1]
  phase2     %state pressure reducing -> phase3 : [alpha>alpha1]
  phase3 -> (junction 25)
  (junction 25) -> phase4_1     %state pressure boosting [order 3] : [alpha>A]
  (junction 25) -> phase4_2     %state pressure reducing [order 2] : [alpha<alpha2]
  (junction 25) -> phase4_3 [order 1] : [alpha2<alpha<A]
  phase4_2     %state pressure reducing -> phase4_3 : [alpha>alpha2]
  phase4_1     %state pressure boosting -> phase4_3 : [alpha<A]
  phase4_3 -> phase5     %state pressure boosting : [alpha<alpha2]
  data: alpha input; alpha1 parameter; alpha2 parameter; omegaR input; state output; A parameter; T1 parameter; T2 parameter; sliprate1 input

== stateflow chart TCS_straight/Control logic/Control logic FR/FR ==
  state state_ [group]
    0:pressure boosting of manual
    1:pressure maintaining
    2:pressure reducing
    3:pressure boosting
    Parameter:
    T1 T2
    alpha1\alpha2\sliprate1\A
    Input: alpha\sliprate
    Output:state
  state phase2     %state pressure reducing
    state phase3_1
      en:
      state= 2;
    state phase3_2
      en:
      state= 1;
    (default) -> phase3_1
    phase3_1 -> phase3_2 : after(T1,sec)
    phase3_2 -> phase3_1 : after(T1,sec)
  state phase0
    en:
    state= 0;
  state phase1
    en:
    state= 1;
  state phase4_2     %state pressure reducing
    state phase4_2_1
      en:
      state= 2;
    state phase4_2_2
      en:
      state= 1;
    (default) -> phase4_2_1
    phase4_2_1 -> phase4_2_2 : after(T1,sec)
    phase4_2_2 -> phase4_2_1 : after(T1,sec)
  state phase4_1     %state pressure boosting
    state phase4_1_1
      en:
      state= 3;
    state phase4_1_2
      en:
      state= 1;
    (default) -> phase4_1_1
    phase4_1_1 -> phase4_1_2 : after(T2,sec)
    phase4_1_2 -> phase4_1_1 : after(T2,sec)
  state phase3
    en:
    state= 1;
  state phase4_ 1 2 3: [group]
    路面附着系数识别阶段
  state phase4_3
    en:
    state= 1;
  state phase5     %state pressure boosting
    state phase5_1
      en:
      state= 3;
    state phase5_2
      en:
      state= 1;
    (default) -> phase5_1
    phase5_1 -> phase5_2 : after(T2,sec)
    phase5_2 -> phase5_1 : after(T2,sec)
  state phase5_ [group]
    第一周期结束
  (default) -> phase0
  phase0 -> phase1 : [alpha<alpha1]
      | %开始作用
  phase1 -> phase2     %state pressure reducing : [omegaR<sliprate1]
  phase5     %state pressure boosting -> phase1 : [alpha<alpha1]
  phase2     %state pressure reducing -> phase3 : [alpha>alpha1]
  phase3 -> (junction 25)
  (junction 25) -> phase4_1     %state pressure boosting [order 3] : [alpha>A]
  (junction 25) -> phase4_2     %state pressure reducing [order 2] : [alpha<alpha2]
  (junction 25) -> phase4_3 [order 1] : [alpha2<alpha<A]
  phase4_2     %state pressure reducing -> phase4_3 : [alpha>alpha2]
  phase4_1     %state pressure boosting -> phase4_3 : [alpha<A]
  phase4_3 -> phase5     %state pressure boosting : [alpha<alpha2]
  data: alpha input; alpha1 parameter; alpha2 parameter; omegaR input; state output; A parameter; T1 parameter; T2 parameter; sliprate1 input

== stateflow chart TCS_straight/Execution phase/Execution phaseF/Execution phaseFR ==
  state state_ [group]
    人工增压0:Inlet = 0,Outlet = 0,Pume = 0;
    保压1:Inlet = 1,Outlet = 0,Pump = 0;
    减压2:Inlet = 1,Outlet = 1,Pump = 1;
    增压3:Inlet = 0,Outlet = 0,Pump = 1.
  state Execution
    state state1
      en:
      %Inlet = 0
      %Outlet = 0
      Pump = 100;
    state state2
      en:
      %Inlet = 1
      %Outlet = 0
      Pump = 300;
    state state3
      en:
      %Inlet = 1
      %Outlet = 1
      Pump = 200;
    state state4
      en:
      %Inlet = 0
      %Outlet = 0
      Pump = 700;
    Execution -> state1 [order 1] : [state == 0]
    Execution -> state2 [order 2] : [state == 1]
    Execution -> state3 [order 3] : [state == 2]
    Execution -> state4 [order 4] : [state == 3]
    (default) -> state1
  (default) -> Execution
  data: state input; Pump output

== stateflow chart TCS_straight/Execution phase/Execution phaseF/Execution phaseFL ==
  state state_ [group]
    人工增压0:Inlet = 0,Outlet = 0,Pume = 0;
    保压1:Inlet = 1,Outlet = 0,Pump = 0;
    减压2:Inlet = 1,Outlet = 1,Pump = 1;
    增压3:Inlet = 0,Outlet = 0,Pump = 1.
  state Execution
    state state1
      en:
      %Inlet = 0
      %Outlet = 0
      Pump = 100;
    state state2
      en:
      %Inlet = 1
      %Outlet = 0
      Pump = 300;
    state state3
      en:
      %Inlet = 1
      %Outlet = 1
      Pump = 200;
    state state4
      en:
      %Inlet = 0
      %Outlet = 0
      Pump = 700;
    Execution -> state1 [order 1] : [state == 0]
    Execution -> state2 [order 2] : [state == 1]
    Execution -> state3 [order 3] : [state == 2]
    Execution -> state4 [order 4] : [state == 3]
    (default) -> state1
  (default) -> Execution
  data: state input; Pump output

== stateflow chart TCS_straight/Execution phase/Execution phaseR/Execution phaseRL ==
  state state_ [group]
    人工增压0:Inlet = 0,Outlet = 0,Pume = 0;
    保压1:Inlet = 1,Outlet = 0,Pump = 0;
    减压2:Inlet = 1,Outlet = 1,Pump = 1;
    增压3:Inlet = 0,Outlet = 0,Pump = 1.
  state Execution
    state state1
      en:
      %Inlet = 0
      %Outlet = 0
      Pump =100;
    state state2
      en:
      %Inlet = 1
      %Outlet = 0
      Pump = 300;
    state state3
      en:
      %Inlet = 1
      %Outlet = 1
      Pump = 200;
    state state4
      en:
      %Inlet = 0
      %Outlet = 0
      Pump = 700;
    Execution -> state1 [order 1] : [state == 0]
    Execution -> state2 [order 2] : [state == 1]
    Execution -> state3 [order 3] : [state == 2]
    Execution -> state4 [order 4] : [state == 3]
    (default) -> state1
  (default) -> Execution
  data: state input; Pump output

== stateflow chart TCS_straight/Execution phase/Execution phaseR/Execution phaseRR ==
  state state_ [group]
    人工增压0:Inlet = 0,Outlet = 0,Pump = 0;
    保压1:Inlet = 1,Outlet = 0,Pump = 0;
    减压2:Inlet = 1,Outlet = 1,Pump = 1;
    增压3:Inlet = 0,Outlet = 0,Pump = 1.
  state Execution
    state state1
      en:
      %Inlet = 0
      %Outlet = 0
      Pump = 100;
    state state2
      en:
      %Inlet = 1
      %Outlet = 0
      Pump =300;
    state state3
      en:
      %Inlet = 1
      %Outlet = 1
      Pump = 200;
    state state4
      en:
      %Inlet = 0
      %Outlet = 0
      Pump = 700;
    Execution -> state1 [order 1] : [state == 0]
    Execution -> state2 [order 2] : [state == 1]
    Execution -> state3 [order 3] : [state == 2]
    Execution -> state4 [order 4] : [state == 3]
    (default) -> state1
  (default) -> Execution
  data: state input; Pump output

== stateflow chart TCS_straight/Control logic/straight control/Chart ==
  state state_ [group]
    0:pressure boosting of manual
    1:pressure maintaining
    2:pressure reducing
    3:pressure boosting
    Parameter:
    T1 T2
    alpha0\Vth
    Input: alpha\sliprate
    Output:state
  state phase1
    en:
    state= 0;
  state phase2
    en:
    state= 0;
  state phase3
    en:
    state= 0;
  state phase5
    en:
    state= 3;
  state phase7
    en:
    state= 0;
  state phase8
    en:
    state= 1;
  state phase02
    en:
    state= 0;
  state phase4
    en:
    state= 0;
  state phase9
    en:
    state= 2;
  state phase6
    en:
    state= 0;
  phase8 -> phase1 : [V_H<Vta]
  (default) -> phase1
  phase1 -> phase2 [order 1] : [Vs<Vth]
      | %开始作用
  phase2 -> phase3 [order 1] : [V_H>=Vta]
  phase3 -> phase5 [order 1] : [V_H>=Vtb]
  phase5 -> phase7 : [a_H<=0]
  phase7 -> phase8 [order 1] : [V_H>=Vtb]
  phase1 -> phase02 [order 2] : [Vs>=Vth]
  phase3 -> phase6 [order 2] : [V_H<Vtb]
  phase2 -> phase4 [order 2] : [V_H<Vta]
  phase7 -> phase9 [order 2] : [V_H<Vtb]
  phase9 -> phase1 : [V_H<Vta]
  phase6 -> phase5 : [a_H>alpha0]
  data: a_H input; Vta input; Vtb input; V_H input; Vs input; Vth input; state output; alpha0 input
